simulink model "simulation_project_A"  (R2024b)
settings: Solver=ode4  StartTime=0.0  StopTime=tend  FixedStep=0.1  MaxStep=0.01  RelTol=1e-6  AbsTol=1e-9
values from neighbouring files (symbols this model uses):
  Cm = 12    [project_A.m]
  E_An = -60    [project_A.m]
  Em0 = -70    [project_A.m]
  g_An = 0.18    [project_A.m]
  gNa_const = input('Insert a value for the constant sodium conductance: \n')    [project_A.m]
  hinf0 = alpha_h0/(alpha_h0+beta_h0)    [project_A.m]
  minf0 = alpha_m0/(alpha_m0+beta_m0)    [project_A.m]
settings Model: Creator=asiarossi  LastModifiedBy=asiarossi
settings SolverCC: ODENIntegrationMethod=ode4
settings DataIOCC: SaveFormat=Array  SaveOutput=off  SignalLogging=off  DSMLogging=off  ReturnWorkspaceOutputs=off

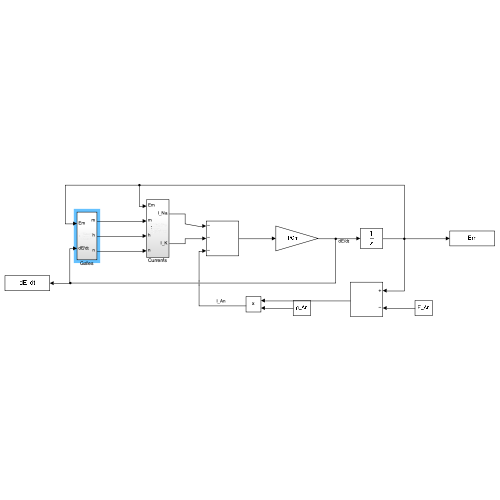
[thumbnail: Simulink's stored preview of the top-level diagram]
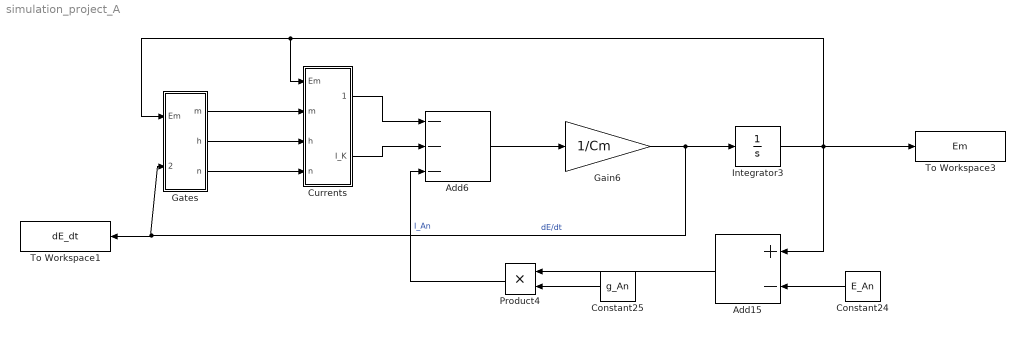
== system simulation_project_A ==
  Add15 : Sum  Inputs=+-
  Add6 : Sum  Inputs=---
  Constant24 : Constant  Value=E_An
  Constant25 : Constant  Value=g_An
  Currents : Subsystem
  Gain6 : Gain  Gain=1/Cm
  Gates : Subsystem
  Integrator3 : Integrator  InitialCondition=Em0
  Product4 : Product
  To Workspace1 : ToWorkspace  VariableName=dE_dt  SampleTime=-1
  To Workspace3 : ToWorkspace  VariableName=Em  SampleTime=-1
  wires:
  Add6/1 -> Gain6/1
  Gain6/1 -> To Workspace1/1, Gates/2(dE/dt), Integrator3/1  "dE/dt"
  Integrator3/1 -> Add15/1, Currents/1(Em), Gates/1(Em), To Workspace3/1
  Add15/1 -> Product4/1
  Constant25/1 -> Product4/2
  Constant24/1 -> Add15/2
  Product4/1 -> Add6/3  "I_An"
  Gates/1(m) -> Currents/2(m)
  Gates/2(h) -> Currents/3(h)
  Gates/3(n) -> Currents/4(n)
  Currents/1(I_Na) -> Add6/1
  Currents/2(I_K) -> Add6/2

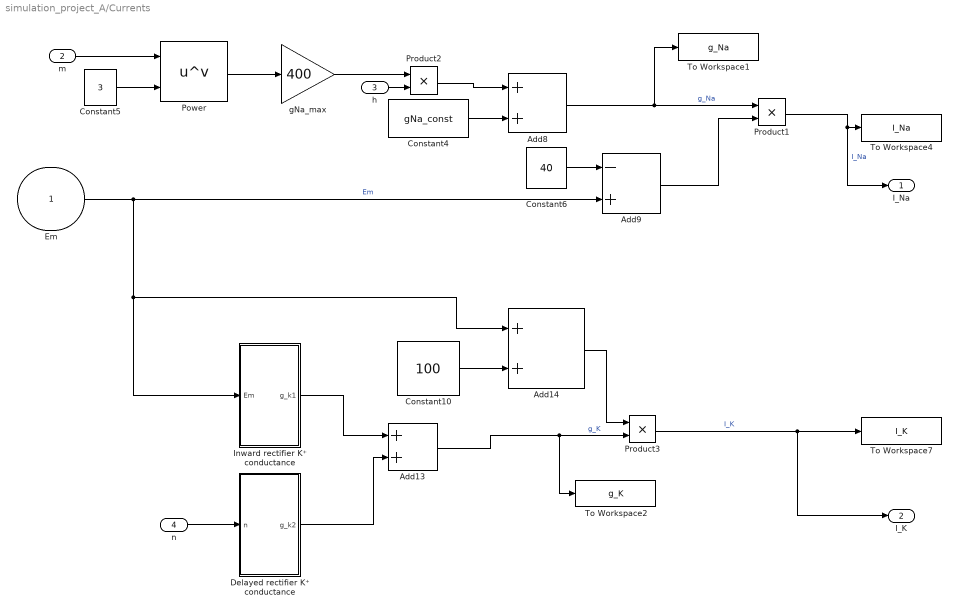
== system simulation_project_A/Currents ==
  Em : Inport
  m : Inport  Port=2
  h : Inport  Port=3
  n : Inport  Port=4
  Add13 : Sum
  Add14 : Sum
  Add8 : Sum
  Add9 : Sum  Inputs=-+
  Constant10 : Constant  Value=100
  Constant4 : Constant  Value=gNa_const
  Constant5 : Constant  Value=3
  Constant6 : Constant  Value=40
  Delayed rectifier K⁺ conductance : Subsystem
  Inward rectifier K⁺ conductance : Subsystem
  Power : Math  Operator=pow
  Product1 : Product
  Product2 : Product
  Product3 : Product
  To Workspace1 : ToWorkspace  VariableName=g_Na  SampleTime=-1
  To Workspace2 : ToWorkspace  VariableName=g_K  SampleTime=-1
  To Workspace4 : ToWorkspace  VariableName=I_Na  SampleTime=-1
  To Workspace7 : ToWorkspace  VariableName=I_K  SampleTime=-1
  gNa_max : Gain  Gain=400
  I_Na : Outport
  I_K : Outport  Port=2
  wires:
  Product2/1 -> Add8/1
  Delayed rectifier K⁺ conductance/1(g_k2) -> Add13/2
  n/1 -> Delayed rectifier K⁺ conductance/1(n)
  Constant6/1 -> Add9/1
  gNa_max/1 -> Product2/1
  Constant4/1 -> Add8/2
  h/1 -> Product2/2
  Add8/1 -> To Workspace1/1, Product1/1  "g_Na"
  Add13/1 -> To Workspace2/1, Product3/2  "g_K"
  m/1 -> Power/1
  Product1/1 -> I_Na/1, To Workspace4/1  "I_Na"
  Product3/1 -> I_K/1, To Workspace7/1  "I_K"
  Add14/1 -> Product3/1
  Constant5/1 -> Power/2
  Power/1 -> gNa_max/1
  Inward rectifier K⁺ conductance/1(g_k1) -> Add13/1
  Constant10/1 -> Add14/2
  Add9/1 -> Product1/2
  Em/1 -> Inward rectifier K⁺ conductance/1(Em), Add14/1, Add9/2  "Em"

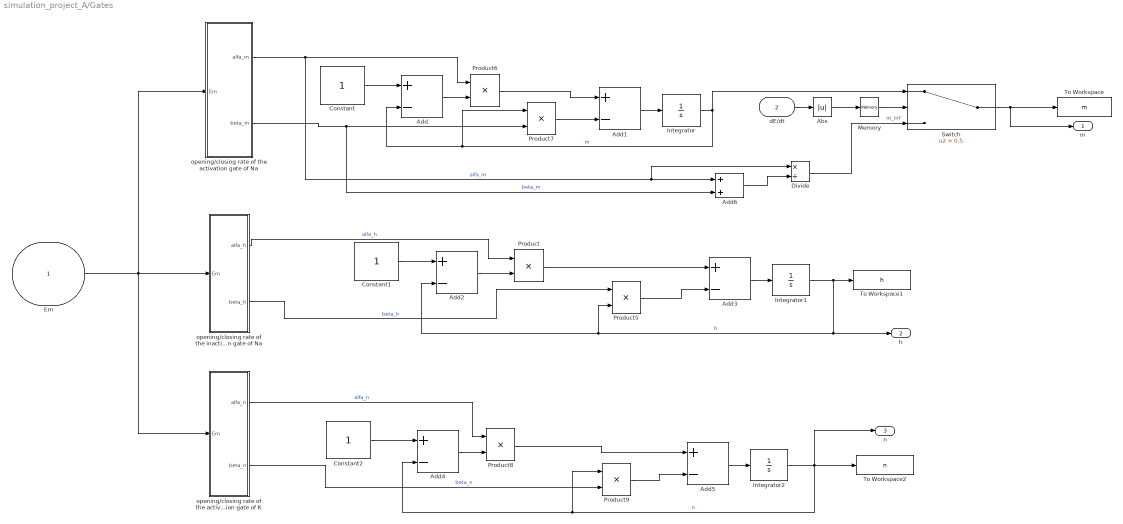
== system simulation_project_A/Gates ==
  Em : Inport
  dE/dt : Inport  Port=2
  Abs : Abs  SaturateOnIntegerOverflow=off
  Add{,1..5} (6 alike) : Sum  Inputs=+-
  Add6 : Sum
  Constant : Constant
  Constant1 : Constant
  Constant2 : Constant
  Divide : Product  Inputs=*/
  Integrator : Integrator  InitialCondition=minf0
  Integrator1 : Integrator  InitialCondition=hinf0
  Integrator2 : Integrator  InitialCondition=0.3
  Memory : Memory
  Product{,5..9} (6 alike) : Product
  Switch : Switch  Criteria=u2 > Threshold  Threshold=0.5  SaturateOnIntegerOverflow=off  InputSameDT=off
  To Workspace : ToWorkspace  VariableName=m  SampleTime=-1
  To Workspace1 : ToWorkspace  VariableName=h  SampleTime=-1
  To Workspace2 : ToWorkspace  VariableName=n  SampleTime=-1
  "opening/closing rate of the activation gate of K " : Subsystem
  opening/closing rate of the activation gate of Na : Subsystem
  opening/closing rate of the inactivation gate of Na : Subsystem
  m : Outport
  h : Outport  Port=2
  n : Outport  Port=3
  wires:
  Em/1 -> opening/closing rate of the activation gate of Na/1(Em), opening/closing rate of the inactivation gate of Na/1(Em), "opening/closing rate of the activation gate of K "/1(Em)
  "opening/closing rate of the activation gate of K "/2(beta_n) -> Product9/2  "beta_n"
  opening/closing rate of the activation gate of Na/1(alfa_m) -> Product6/1, Divide/1, Add6/1  "alfa_m"
  Add/1 -> Product6/2
  Product8/1 -> Add5/1
  Add3/1 -> Integrator1/1
  Product9/1 -> Add5/2
  Product6/1 -> Add1/1
  Constant2/1 -> Add4/1
  opening/closing rate of the inactivation gate of Na/2(beta_h) -> Product5/1  "beta_h"
  Product7/1 -> Add1/2
  Product5/1 -> Add3/2
  Add4/1 -> Product8/2
  Product/1 -> Add3/1
  Integrator1/1 -> h/1, Product5/2, Add2/2, To Workspace1/1  "h"
  Integrator2/1 -> n/1, Product9/1, Add4/2, To Workspace2/1  "n"
  Constant1/1 -> Add2/1
  "opening/closing rate of the activation gate of K "/1(alfa_n) -> Product8/1  "alfa_n"
  Add5/1 -> Integrator2/1
  Add2/1 -> Product/2
  Add1/1 -> Integrator/1
  Constant/1 -> Add/1
  opening/closing rate of the inactivation gate of Na/1(alfa_h) -> Product/1  "alfa_h"
  opening/closing rate of the activation gate of Na/2(beta_m) -> Add6/2, Product7/2  "beta_m"
  Integrator/1 -> Product7/1, Add/2, Switch/1  "m"
  dE/dt/1 -> Abs/1
  Abs/1 -> Memory/1
  Memory/1 -> Switch/2
  Switch/1 -> m/1, To Workspace/1
  Add6/1 -> Divide/2
  Divide/1 -> Switch/3  "m_inf"

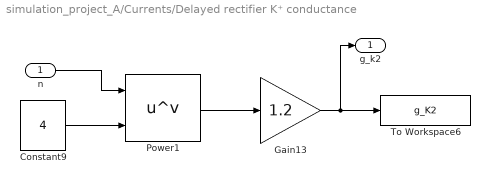
== system simulation_project_A/Currents/Delayed rectifier K⁺ conductance ==
  n : Inport
  Constant9 : Constant  Value=4
  Gain13 : Gain  Gain=1.2
  Power1 : Math  Operator=pow
  To Workspace6 : ToWorkspace  VariableName=g_K2  SampleTime=-1
  g_k2 : Outport
  wires:
  n/1 -> Power1/1
  Constant9/1 -> Power1/2
  Gain13/1 -> g_k2/1, To Workspace6/1
  Power1/1 -> Gain13/1

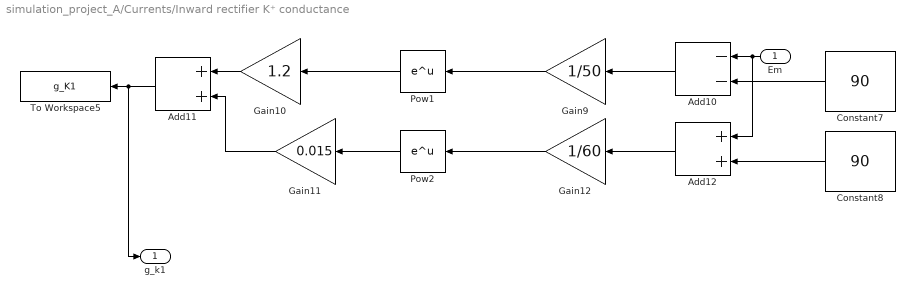
== system simulation_project_A/Currents/Inward rectifier K⁺ conductance ==
  Em : Inport
  Add10 : Sum  Inputs=--
  Add11 : Sum
  Add12 : Sum
  Constant7 : Constant  Value=90
  Constant8 : Constant  Value=90
  Gain10 : Gain  Gain=1.2
  Gain11 : Gain  Gain=0.015
  Gain12 : Gain  Gain=1/60
  Gain9 : Gain  Gain=1/50
  Pow1 : Math  SignedPower=on  RndMeth=Zero
  Pow2 : Math  SignedPower=on  RndMeth=Zero
  To Workspace5 : ToWorkspace  VariableName=g_K1  SampleTime=-1
  g_k1 : Outport
  wires:
  Pow1/1 -> Gain10/1
  Pow2/1 -> Gain11/1
  Add12/1 -> Gain12/1
  Constant7/1 -> Add10/2
  Gain10/1 -> Add11/1
  Gain12/1 -> Pow2/1
  Constant8/1 -> Add12/2
  Add11/1 -> g_k1/1, To Workspace5/1
  Em/1 -> Add12/1, Add10/1
  Gain11/1 -> Add11/2
  Gain9/1 -> Pow1/1
  Add10/1 -> Gain9/1

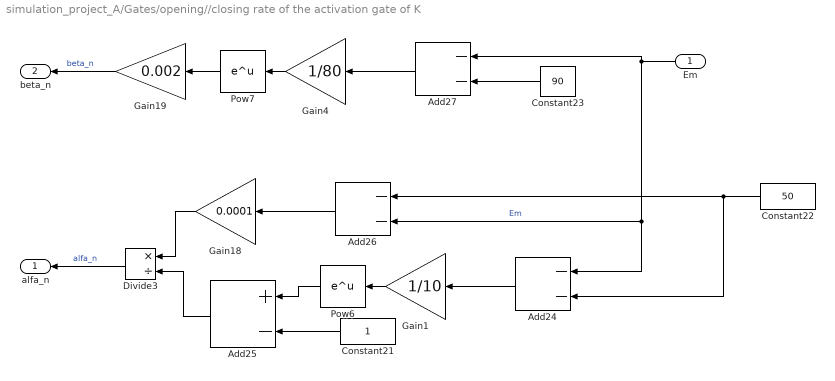
== system simulation_project_A/Gates/opening//closing rate of the activation gate of K  ==
  Em : Inport
  Add24 : Sum  Inputs=--
  Add25 : Sum  Inputs=+-
  Add26 : Sum  Inputs=--
  Add27 : Sum  Inputs=--
  Constant21 : Constant
  Constant22 : Constant  Value=50
  Constant23 : Constant  Value=90
  Divide3 : Product  Inputs=*/
  Gain1 : Gain  Gain=1/10
  Gain18 : Gain  Gain=0.0001
  Gain19 : Gain  Gain=0.002
  Gain4 : Gain  Gain=1/80
  Pow6 : Math  SignedPower=on  RndMeth=Zero
  Pow7 : Math  SignedPower=on  RndMeth=Zero
  alfa_n : Outport
  beta_n : Outport  Port=2
  wires:
  Gain19/1 -> beta_n/1  "beta_n"
  Add24/1 -> Gain1/1
  Constant23/1 -> Add27/2
  Divide3/1 -> alfa_n/1  "alfa_n"
  Gain4/1 -> Pow7/1
  Em/1 -> Add24/1, Add26/2, Add27/1  "Em"
  Add26/1 -> Gain18/1
  Add27/1 -> Gain4/1
  Constant22/1 -> Add24/2, Add26/1
  Pow7/1 -> Gain19/1
  Add25/1 -> Divide3/2
  Gain1/1 -> Pow6/1
  Constant21/1 -> Add25/2
  Gain18/1 -> Divide3/1
  Pow6/1 -> Add25/1

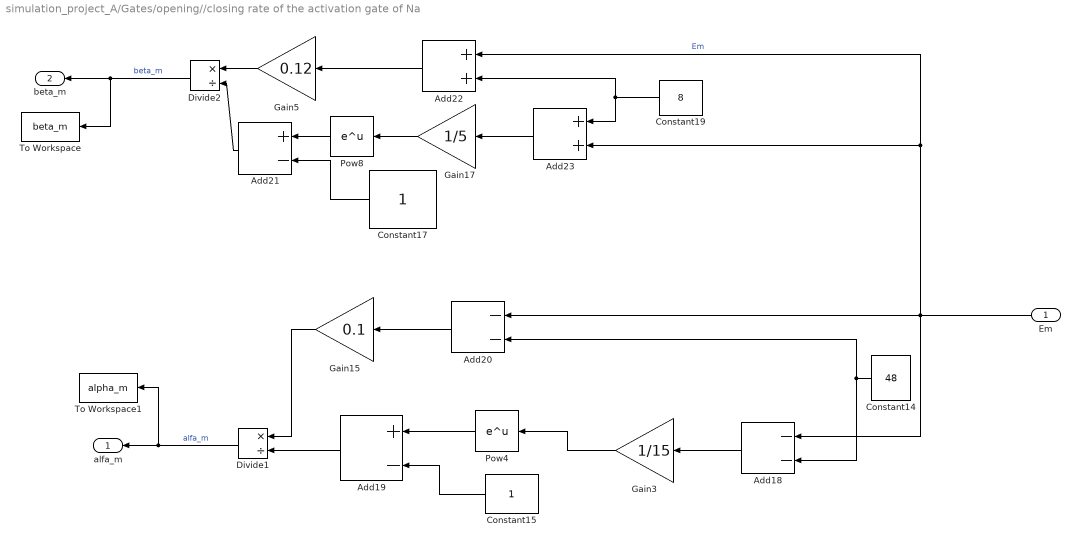
== system simulation_project_A/Gates/opening//closing rate of the activation gate of Na ==
  Em : Inport
  Add18 : Sum  Inputs=--
  Add19 : Sum  Inputs=+-
  Add20 : Sum  Inputs=--
  Add21 : Sum  Inputs=+-
  Add22 : Sum
  Add23 : Sum
  Constant14 : Constant  Value=48
  Constant15 : Constant
  Constant17 : Constant
  Constant19 : Constant  Value=8
  Divide1 : Product  Inputs=*/
  Divide2 : Product  Inputs=*/
  Gain15 : Gain  Gain=0.1
  Gain17 : Gain  Gain=1/5
  Gain3 : Gain  Gain=1/15
  Gain5 : Gain  Gain=0.12
  Pow4 : Math  SignedPower=on  RndMeth=Zero
  Pow8 : Math  SignedPower=on  RndMeth=Zero
  To Workspace : ToWorkspace  VariableName=beta_m  SampleTime=-1
  To Workspace1 : ToWorkspace  VariableName=alpha_m  SampleTime=-1
  alfa_m : Outport
  beta_m : Outport  Port=2
  wires:
  Divide1/1 -> To Workspace1/1, alfa_m/1  "alfa_m"
  Divide2/1 -> To Workspace/1, beta_m/1  "beta_m"
  Add22/1 -> Gain5/1
  Gain5/1 -> Divide2/1
  Pow4/1 -> Add19/1
  Constant14/1 -> Add18/2, Add20/2
  Em/1 -> Add22/1, Add23/2, Add20/1, Add18/1  "Em"
  Add19/1 -> Divide1/2
  Constant19/1 -> Add23/1, Add22/2
  Constant17/1 -> Add21/2
  Add18/1 -> Gain3/1
  Gain15/1 -> Divide1/1
  Add23/1 -> Gain17/1
  Add20/1 -> Gain15/1
  Gain17/1 -> Pow8/1
  Add21/1 -> Divide2/2
  Constant15/1 -> Add19/2
  Pow8/1 -> Add21/1
  Gain3/1 -> Pow4/1

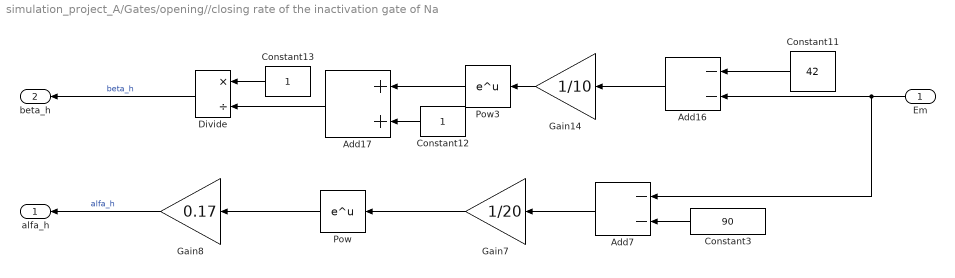
== system simulation_project_A/Gates/opening//closing rate of the inactivation gate of Na ==
  Em : Inport
  Add16 : Sum  Inputs=--
  Add17 : Sum
  Add7 : Sum  Inputs=--
  Constant11 : Constant  Value=42
  Constant12 : Constant
  Constant13 : Constant
  Constant3 : Constant  Value=90
  Divide : Product  Inputs=*/
  Gain14 : Gain  Gain=1/10
  Gain7 : Gain  Gain=1/20
  Gain8 : Gain  Gain=0.17
  Pow : Math  SignedPower=on  RndMeth=Zero
  Pow3 : Math  SignedPower=on  RndMeth=Zero
  alfa_h : Outport
  beta_h : Outport  Port=2
  wires:
  Divide/1 -> beta_h/1  "beta_h"
  Em/1 -> Add7/1, Add16/2
  Constant13/1 -> Divide/1
  Add7/1 -> Gain7/1
  Add17/1 -> Divide/2
  Add16/1 -> Gain14/1
  Constant3/1 -> Add7/2
  Gain7/1 -> Pow/1
  Gain8/1 -> alfa_h/1  "alfa_h"
  Pow/1 -> Gain8/1
  Gain14/1 -> Pow3/1
  Constant11/1 -> Add16/1
  Constant12/1 -> Add17/2
  Pow3/1 -> Add17/1
